simulink model "quadcopter_LQR_test"  (R2015b)
settings: Solver=VariableStepAuto  StartTime=0.0  StopTime=50  RelTol=1e-3
values from neighbouring files (symbols this model uses):
  LQR_D = 0.15    [init_LQR_test.m]    (also in init_LQRi_test.m)
  LQR_I = 0    [init_LQR_test.m]    (also in init_LQRi_test.m)
  LQR_K = 0.17    [init_LQR_test.m]    (also in init_LQRi_test.m)
undefined symbols (not defined in the file or in its folder): euleranglelim, g, innerLoopSampleRate, K, k, m, N, omegalim, seed
libraries: simulink x2
settings Model: Creator=Daniel  LastModifiedBy=mgreiff
settings SolverCC: AlgebraicLoopSolver=LineSearch

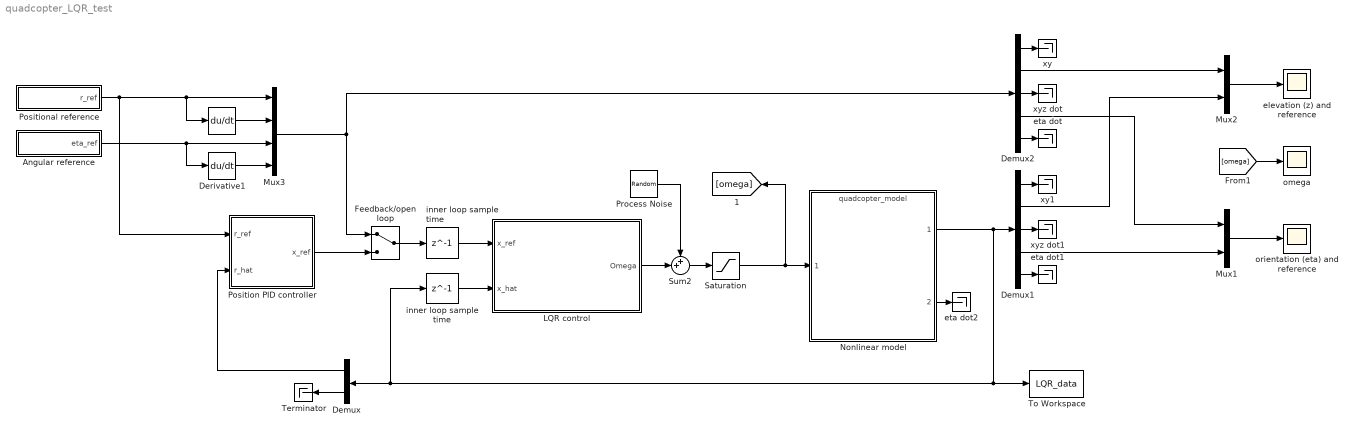
== system quadcopter_LQR_test ==
  "        " : Derivative
  "   eta dot" : Terminator
  "   eta dot1" : Terminator
  "   eta dot2" : Terminator
  "   xy" : Terminator
  "   xy1" : Terminator
  "  xyz dot" : Terminator
  "  xyz dot1" : Terminator
  Angular reference : Subsystem
  Demux : Demux  Outputs=[3,9]
  Demux1 : Demux  Outputs=[2,1,3,3,3]
  Demux2 : Demux  Outputs=[2,1,3,3,3]
  Derivative1 : Derivative
  Feedback/open loop : ManualSwitch
  LQR control : Subsystem
  Mux1 : Mux  Inputs=2
  Mux2 : Mux  Inputs=2
  Mux3 : Mux  Inputs=[3,3,3,3]
  Nonlinear model : ModelReference  ModelNameDialog=quadcopter_model.mdl  SimulationMode=Normal  ModelReferenceVersion=1.117  CopyOfModelName=quadcopter_model.mdl
  Position PID controller : Subsystem
  Positional reference : Subsystem
  Process Noise : RandomNumber  Mean=[0 0 0 0]'  Variance=0  SampleTime=0.01
  Saturation : Saturate  UpperLimit=omegalim(2)  LowerLimit=omegalim(1)
  Sum2 : Sum  Inputs=++|
  Terminator : Terminator
  To Workspace : ToWorkspace  VariableName=LQR_data  SaveFormat=Timeseries  SampleTime=-1
  elevation (z) and reference : Scope
  inner loop sample time : Delay  DelayLength=1  InitialCondition=0  SampleTime=innerLoopSampleRate
  "inner loop sample time " : Delay  DelayLength=1  InitialCondition=0  SampleTime=innerLoopSampleRate
  "omega " : Scope
  orientation (eta) and reference : Scope
  wires:
  Process Noise/1 -> Sum2/1
  Sum2/1 -> Saturation/1
  LQR control/1(Omega) -> Sum2/2
  Demux2/2 -> Mux2/1
  Mux2/1 -> elevation (z) and reference/1
  Demux1/2 -> Mux2/2
  Nonlinear model/1 -> "inner loop sample time "/1, Demux/1, To Workspace/1, Demux1/1
  Mux1/1 -> orientation (eta) and reference/1
  Demux/2 -> Terminator/1
  Demux/1 -> Position PID controller/2(r_hat)
  Angular reference/1(eta_ref) -> Derivative1/1, Mux3/3
  Positional reference/1(r_ref) -> Position PID controller/1(r_ref), Mux3/1, "        "/1
  "        "/1 -> Mux3/2
  Derivative1/1 -> Mux3/4
  Feedback/open loop/1 -> inner loop sample time/1
  Position PID controller/1(x_ref) -> Feedback/open loop/2
  Saturation/1 -> [omega], Nonlinear model/1
  "inner loop sample time "/1 -> LQR control/2(x_hat)
  inner loop sample time/1 -> LQR control/1(x_ref)
  Mux3/1 -> Demux2/1, Feedback/open loop/1
  Demux2/3 -> "  xyz dot"/1
  Demux2/5 -> "   eta dot"/1
  Demux2/1 -> "   xy"/1
  Demux1/3 -> "  xyz dot1"/1
  Demux1/5 -> "   eta dot1"/1
  Demux1/1 -> "   xy1"/1
  Demux1/4 -> Mux1/2
  [omega] -> "omega "/1
  Nonlinear model/2 -> "   eta dot2"/1
  Demux2/4 -> Mux1/1

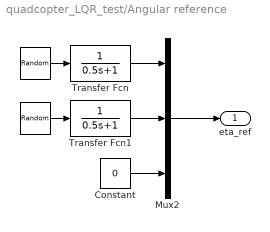
== system quadcopter_LQR_test/Angular reference ==
  " " : UniformRandomNumber  Minimum=-0.2  Maximum=0.2  Seed=4+seed  SampleTime=10
  "   " : UniformRandomNumber  Minimum=-0.2  Maximum=0.2  Seed=3+seed  SampleTime=10
  Constant : Constant  Value=0
  Mux2 : Mux  Inputs=3
  Transfer Fcn : TransferFcn  Denominator=[0.5 1]
  Transfer Fcn1 : TransferFcn  Denominator=[0.5 1]
  eta_ref : Outport
  wires:
  Mux2/1 -> eta_ref/1
  "   "/1 -> Transfer Fcn/1
  " "/1 -> Transfer Fcn1/1
  Transfer Fcn/1 -> Mux2/1
  Transfer Fcn1/1 -> Mux2/2
  Constant/1 -> Mux2/3

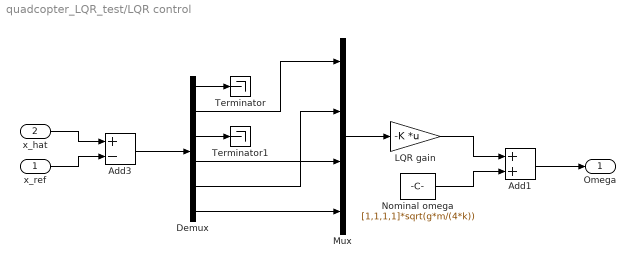
== system quadcopter_LQR_test/LQR control ==
  x_ref : Inport  PortDimensions=12
  x_hat : Inport  Port=2  PortDimensions=12
  Add1 : Sum
  Add3 : Sum  Inputs=+-
  Demux : Demux  Outputs=[2,1,2,1,3,3]
  LQR gain : Gain  Gain=-K  Multiplication=Matrix(K*u)
  Mux : Mux
  Nominal omega : Constant  Value=[1,1,1,1]*sqrt(g*m/(4*k))
  Terminator : Terminator
  Terminator1 : Terminator
  Omega : Outport
  wires:
  Mux/1 -> LQR gain/1
  LQR gain/1 -> Add1/1
  Nominal omega/1 -> Add1/2
  Add1/1 -> Omega/1
  Demux/1 -> Terminator/1
  x_ref/1 -> Add3/2
  x_hat/1 -> Add3/1
  Add3/1 -> Demux/1
  Demux/2 -> Mux/1
  Demux/3 -> Terminator1/1
  Demux/4 -> Mux/3
  Demux/5 -> Mux/2
  Demux/6 -> Mux/4

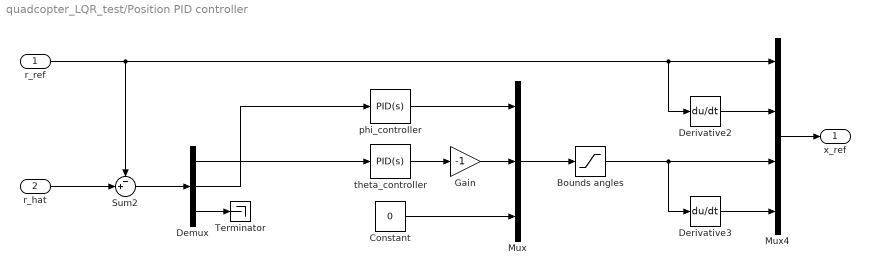
== system quadcopter_LQR_test/Position PID controller ==
  r_ref : Inport
  r_hat : Inport  Port=2
  Bounds angles : Saturate  UpperLimit=euleranglelim(2)  LowerLimit=euleranglelim(1)
  Constant : Constant  Value=0
  Demux : Demux  Outputs=3
  Derivative2 : Derivative
  Derivative3 : Derivative
  Gain : Gain  Gain=-1
  Mux : Mux  Inputs=3
  Mux4 : Mux  Inputs=[3,3,3,3]
  Sum2 : Sum  Inputs=-+|
  Terminator : Terminator
  phi_controller : simulink/Continuous/PID Controller  Controller=PID  TimeDomain=Continuous-time  SampleTime=-1  IntegratorMethod=Forward Euler  FilterMethod=Forward Euler  Form=Parallel  UseFilter=on  ControllerParametersSource=internal  P=LQR_K  I=LQR_I  D=LQR_D  N=N  InitialConditionSource=internal  InitialConditionForIntegrator=0  InitialConditionForFilter=0  ExternalReset=none  LimitOutput=off  UpperSaturationLimit=inf  LowerSaturationLimit=-inf  LinearizeAsGain=on  AntiWindupMode=none  Kb=1  TrackingMode=off  Kt=1  PParamMin=[]  PParamMax=[]  IParamMin=[]  IParamMax=[]  DParamMin=[]  DParamMax=[]  NParamMin=[]  NParamMax=[]  KbParamMin=[]  KbParamMax=[]  KtParamMin=[]  KtParamMax=[]  POutMin=[]  POutMax=[]  IOutMin=[]  IOutMax=[]  DOutMin=[]  DOutMax=[]  NOutMin=[]  NOutMax=[]  KbOutMin=[]  KbOutMax=[]  KtOutMin=[]  KtOutMax=[]  IntegratorOutMin=[]  IntegratorOutMax=[]  FilterOutMin=[]  FilterOutMax=[]  SumOutMin=[]  SumOutMax=[]  SumI1OutMin=[]  SumI1OutMax=[]  SumI2OutMin=[]  SumI2OutMax=[]  SumI3OutMin=[]  SumI3OutMax=[]  SumDOutMin=[]  SumDOutMax=[]  SaturationOutMin=[]  SaturationOutMax=[]  IntegratorContinuousStateAttributes=''  IntegratorStateMustResolveToSignalObject=off  IntegratorRTWStateStorageClass=Auto  FilterContinuousStateAttributes=''  FilterStateMustResolveToSignalObject=off  FilterRTWStateStorageClass=Auto  DifferentiatorICPrevScaledInput=0  DifferentiatorOutMin=[]  DifferentiatorOutMax=[]
  theta_controller : simulink/Continuous/PID Controller  Controller=PID  TimeDomain=Continuous-time  SampleTime=-1  IntegratorMethod=Forward Euler  FilterMethod=Forward Euler  Form=Parallel  UseFilter=on  ControllerParametersSource=internal  P=LQR_K  I=LQR_I  D=LQR_D  N=N  InitialConditionSource=internal  InitialConditionForIntegrator=0  InitialConditionForFilter=0  ExternalReset=none  LimitOutput=off  UpperSaturationLimit=inf  LowerSaturationLimit=-inf  LinearizeAsGain=on  AntiWindupMode=none  Kb=1  TrackingMode=off  Kt=1  PParamMin=[]  PParamMax=[]  IParamMin=[]  IParamMax=[]  DParamMin=[]  DParamMax=[]  NParamMin=[]  NParamMax=[]  KbParamMin=[]  KbParamMax=[]  KtParamMin=[]  KtParamMax=[]  POutMin=[]  POutMax=[]  IOutMin=[]  IOutMax=[]  DOutMin=[]  DOutMax=[]  NOutMin=[]  NOutMax=[]  KbOutMin=[]  KbOutMax=[]  KtOutMin=[]  KtOutMax=[]  IntegratorOutMin=[]  IntegratorOutMax=[]  FilterOutMin=[]  FilterOutMax=[]  SumOutMin=[]  SumOutMax=[]  SumI1OutMin=[]  SumI1OutMax=[]  SumI2OutMin=[]  SumI2OutMax=[]  SumI3OutMin=[]  SumI3OutMax=[]  SumDOutMin=[]  SumDOutMax=[]  SaturationOutMin=[]  SaturationOutMax=[]  IntegratorContinuousStateAttributes=''  IntegratorStateMustResolveToSignalObject=off  IntegratorRTWStateStorageClass=Auto  FilterContinuousStateAttributes=''  FilterStateMustResolveToSignalObject=off  FilterRTWStateStorageClass=Auto  DifferentiatorICPrevScaledInput=0  DifferentiatorOutMin=[]  DifferentiatorOutMax=[]
  x_ref : Outport
  wires:
  Constant/1 -> Mux/3
  theta_controller/1 -> Gain/1
  phi_controller/1 -> Mux/1
  Demux/3 -> Terminator/1
  Demux/1 -> theta_controller/1
  Demux/2 -> phi_controller/1
  Gain/1 -> Mux/2
  Mux/1 -> Bounds angles/1
  r_hat/1 -> Sum2/2
  Sum2/1 -> Demux/1
  Bounds angles/1 -> Derivative3/1, Mux4/3
  r_ref/1 -> Sum2/1, Derivative2/1, Mux4/1
  Derivative2/1 -> Mux4/2
  Derivative3/1 -> Mux4/4
  Mux4/1 -> x_ref/1

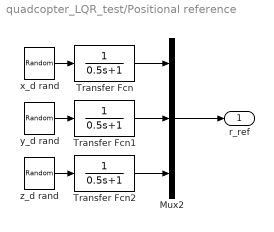
== system quadcopter_LQR_test/Positional reference ==
  Mux2 : Mux  Inputs=3
  Transfer Fcn : TransferFcn  Denominator=[0.5 1]
  Transfer Fcn1 : TransferFcn  Denominator=[0.5 1]
  Transfer Fcn2 : TransferFcn  Denominator=[0.5 1]
  x_d rand : UniformRandomNumber  Minimum=-30  Maximum=30  Seed=0+seed  SampleTime=10
  y_d rand : UniformRandomNumber  Minimum=-30  Maximum=30  Seed=1+seed  SampleTime=10
  z_d rand : UniformRandomNumber  Minimum=0  Maximum=15  Seed=2+seed  SampleTime=10
  r_ref : Outport
  wires:
  Mux2/1 -> r_ref/1
  x_d rand/1 -> Transfer Fcn/1
  y_d rand/1 -> Transfer Fcn1/1
  z_d rand/1 -> Transfer Fcn2/1
  Transfer Fcn/1 -> Mux2/1
  Transfer Fcn1/1 -> Mux2/2
  Transfer Fcn2/1 -> Mux2/3
